simulink model "VMD"  (R2018a)
settings: configuration reference "cs_ert" (kept outside this file)
settings Model: DataDictionary=VMD.sldd  Creator=zhoutinglin  LastModifiedBy=zhoutinglin

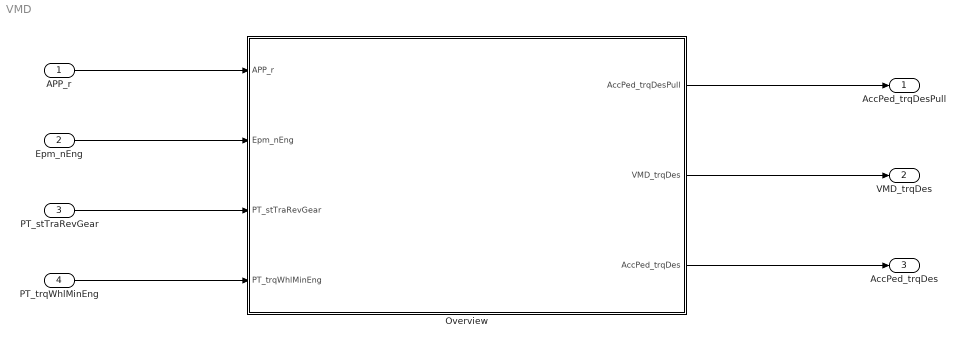
== system VMD ==
  APP_r : Inport
  Epm_nEng : Inport  Port=2
  PT_stTraRevGear : Inport  Port=3
  PT_trqWhlMinEng : Inport  Port=4
  Overview : Subsystem
  AccPed_trqDesPull : Outport
  VMD_trqDes : Outport  Port=2
  AccPed_trqDes : Outport  Port=3
  wires:
  APP_r/1 -> Overview/1(APP_r)
  Epm_nEng/1 -> Overview/2(Epm_nEng)
  PT_stTraRevGear/1 -> Overview/3(PT_stTraRevGear)
  PT_trqWhlMinEng/1 -> Overview/4(PT_trqWhlMinEng)
  Overview/1(AccPed_trqDesPull) -> AccPed_trqDesPull/1
  Overview/2(VMD_trqDes) -> VMD_trqDes/1
  Overview/3(AccPed_trqDes) -> AccPed_trqDes/1

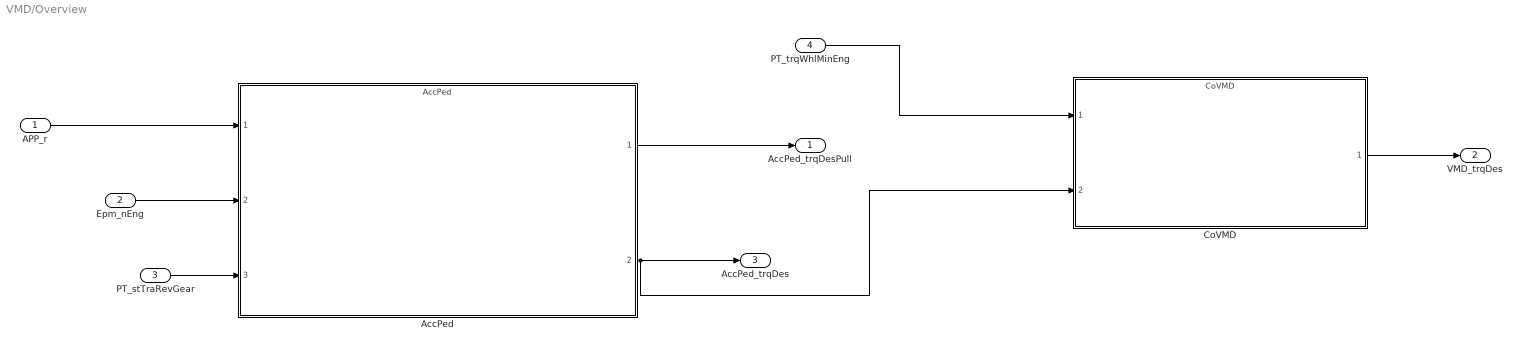
== system VMD/Overview ==
  APP_r : Inport
  Epm_nEng : Inport  Port=2
  PT_stTraRevGear : Inport  Port=3
  PT_trqWhlMinEng : Inport  Port=4
  AccPed : ModelReference  ModelNameDialog=AccPed  SimulationMode=Normal  ModelReferenceVersion=1.5
  CoVMD : ModelReference  ModelNameDialog=CoVMD  SimulationMode=Normal  ModelReferenceVersion=1.5
  AccPed_trqDesPull : Outport
  VMD_trqDes : Outport  Port=2
  AccPed_trqDes : Outport  Port=3
  wires:
  APP_r/1 -> AccPed/1
  Epm_nEng/1 -> AccPed/2
  PT_stTraRevGear/1 -> AccPed/3
  PT_trqWhlMinEng/1 -> CoVMD/1
  AccPed/1 -> AccPed_trqDesPull/1
  AccPed/2 -> CoVMD/2, AccPed_trqDes/1
  CoVMD/1 -> VMD_trqDes/1
